simulink model "Use_Cases_N1_b"  (R2020b)
settings: Solver=ode3  StartTime=0.0  StopTime=inf  FixedStep=0.05  RelTol=1e-3
libraries: simulink x1, Utilities x1, XBotBlockToolbox x1

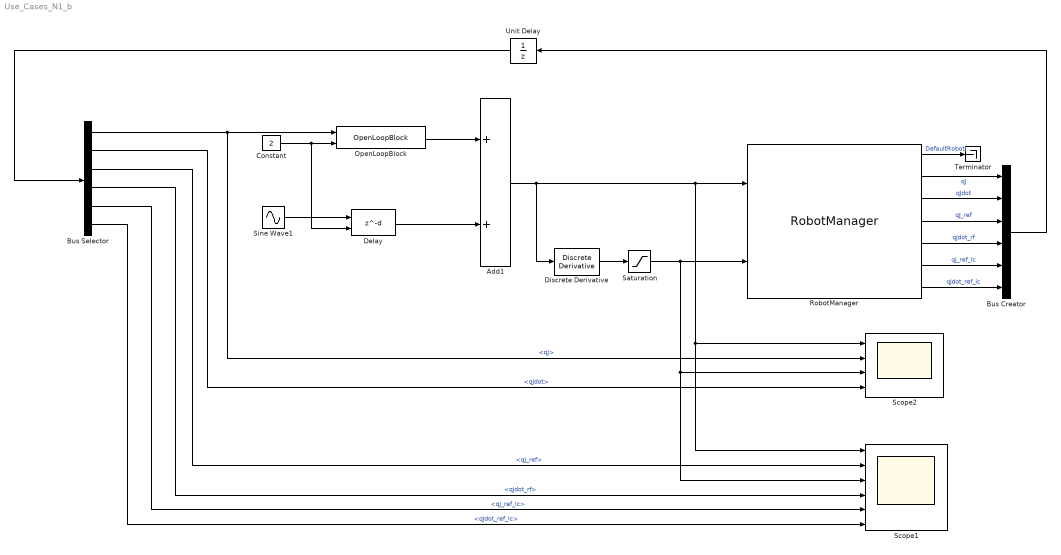
== system Use_Cases_N1_b ==
  Add1 : Sum
  Bus Creator : BusCreator  Inputs=6
  Bus Selector : BusSelector  OutputSignals=qJ,qJdot,qJ_ref,qJdot_rf,qJ_ref_lc,qJdot_ref_lc
  Constant : Constant  Value=2
  Delay : Delay  DelayLengthSource=Input port  DelayLength=1  InitialCondition=0
  Discrete Derivative : simulink/Discrete/Discrete Derivative  gainval=1.0  ICPrevScaledInput=0.0  OutMin=[]  OutMax=[]  OutDataType=fixdt(1, 16)  OutScaling=2^-10  DoSatur=off
  OpenLoopBlock : Utilities/OpenLoopBlock  SystemSampleTime=-1  VariantActivationTime=update diagram  Latency=0  AutoFrameSizeCalculation=off
  RobotManager : XBotBlockToolbox/RobotManager  RobotName=DefaultRobot  ModelName=DefaultRobot  UseExtRobot=Off  SyncWithModel=Off  ReadingsList={ 'qJ', 'qJdot', 'qJ_ref', 'qJdot_ref' }  MechanicalLimitsList={}  MechanicalLimitsCheck=On  MechanicalLimitsEnforce=On  SensorList={}  ReferencesList={ 'qJ_ref', 'qJdot_ref' }  OldRobotName=DefaultRobot
  Saturation : Saturate  UpperLimit=0.2  LowerLimit=-0.2
  Scope1 : Scope  NumInputPorts=6
  Scope2 : Scope  NumInputPorts=4
  Sine Wave1 : Sin  Amplitude=0.2  SampleTime=0
  Terminator : Terminator
  Unit Delay : UnitDelay  SampleTime=-1  HasFrameUpgradeWarning=on
  wires:
  Bus Selector/2 -> Scope2/4  "<qJdot>"
  Add1/1 -> Discrete Derivative/1, Scope1/1, Scope2/1, RobotManager/1
  Discrete Derivative/1 -> Saturation/1
  Saturation/1 -> Scope1/3, Scope2/3, RobotManager/2
  Bus Selector/1 -> Scope2/2, OpenLoopBlock/1  "<qJ>"
  OpenLoopBlock/1 -> Add1/1
  Bus Selector/3 -> Scope1/2  "<qJ_ref>"
  Bus Selector/4 -> Scope1/4  "<qJdot_rf>"
  RobotManager/1 -> Terminator/1  "DefaultRobot"
  RobotManager/2 -> Bus Creator/1  "qJ"
  RobotManager/3 -> Bus Creator/2  "qJdot"
  RobotManager/4 -> Bus Creator/3  "qJ_ref"
  RobotManager/5 -> Bus Creator/4  "qJdot_rf"
  Bus Creator/1 -> Unit Delay/1
  Unit Delay/1 -> Bus Selector/1
  Constant/1 -> Delay/2, OpenLoopBlock/2
  RobotManager/6 -> Bus Creator/5  "qJ_ref_lc"
  RobotManager/7 -> Bus Creator/6  "qJdot_ref_lc"
  Bus Selector/5 -> Scope1/5  "<qJ_ref_lc>"
  Bus Selector/6 -> Scope1/6  "<qJdot_ref_lc>"
  Sine Wave1/1 -> Delay/1
  Delay/1 -> Add1/2
